simulink model "ImageTest"  (R2015b)
settings: Solver=VariableStepAuto  StartTime=0.0  StopTime=10.0  RelTol=1e-3
undefined symbols (not defined in the file): gray
libraries: visionconversions x1, visionstatistics x1, dspvision x1, visionsinks x1, simulink x1
settings Model: Creator=henry  LastModifiedBy=henry

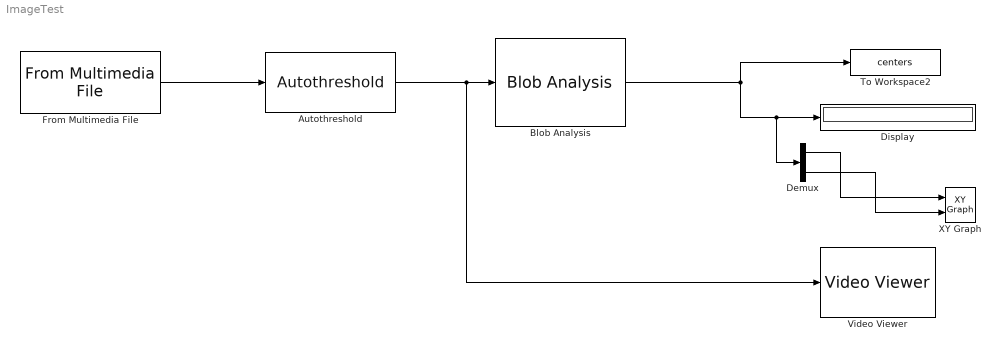
== system ImageTest ==
  Autothreshold : visionconversions/Autothreshold  operator=>  threshOut=off  effMetricOut=off  userDefinedRange=off  umin=0  umax=255  outOfRngOpt=Warn and saturate  scaleThreshold=off  scaleFactor=1  P1Mode=Specify word length  P1WordLength=32  P1FracLength=30  P2Mode=Specify word length  P2WordLength=32  P2FracLength=22  P3Mode=Specify word length  P3WordLength=32  P3FracLength=14  P4Mode=Binary point scaling  P4WordLength=32  P4FracLength=15  Q1Mode=Specify word length  Q1WordLength=32  Q1FracLength=16  EMMode=Specify word length  EMWordLength=16  EMFracLength=14  roundingMode=Floor  overflowMode=off
  Blob Analysis : visionstatistics/Blob Analysis  Tag=vipblks_row_conv  area=off  centroid=on  bBox=off  majorAxis=off  minorAxis=off  angle=off  eccentricity=off  equivDiameterSq=off  extent=off  perimeter=off  maxBlobs=1  warnIfNumBlobsExceeded=off  isCount=off  useMinArea=on  minArea=2000  useMaxArea=on  maxArea=3000  excludeBorderBlob=on  outDT=double  isOutVarDim=off  isFill=off  fillValues=-1  conn=8  isLabel=off  outputMode=Binary point scaling  outputWordLength=32  outputFracLength=16  firstCoeffMode=Binary point scaling  firstCoeffWordLength=16  firstCoeffFracLength=14  secondCoeffMode=Binary point scaling  secondCoeffWordLength=32  secondCoeffFracLength=16  accumMode=Binary point scaling  accumWordLength=32  accumFracLength=0  prodOutputMode=Binary point scaling  prodOutputWordLength=32  prodOutputFracLength=16  roundingMode=Floor  overflowMode=off
  Demux : Demux  Outputs=2
  Display : Display
  From Multimedia File : dspvision/From Multimedia File  inputFilename=/home/henry/MatLab Homework/UH Special Topics/Gitup/MagneticController/Test Videos/output3.ogg  loop=on  numPlays=inf  outputStreams=Video only  videoDataType=single  audioDataType=int16  inheritSampleTime=on  userDefinedSampleTime=1/30  noAudioOutput=off  isIntensityVideo=off  fourcc=Intensity  colorVideoFormat=One multidimensional signal  outputEOF=off  dataOrg=Column-major  audioFrameSize=1024  computeAudioFrameSize=off  outSamplingMode=Sample based
  To Workspace2 : ToWorkspace  VariableName=centers  SampleTime=-1
  Video Viewer : visionsinks/Video Viewer  inputType=Obsolete7b  imagePorts=One multidimensional signal  useColorMap=off  colormapValue=gray(256)  specRange=off  minInputVal=0  maxInputVal=255  FigPos=[181 716 975 554]  AxisZoom=on  trueSizedOnce=off  OpenAtMdlStart=on  DefaultConfigurationName=vipscopes.VideoViewerScopeCfg
  XY Graph : simulink/Sinks/XY Graph  xmin=0  xmax=700  ymin=0  ymax=700  st=-1
  wires:
  Autothreshold/1 -> Video Viewer/1, Blob Analysis/1
  Blob Analysis/1 -> To Workspace2/1, Demux/1, Display/1
  Demux/1 -> XY Graph/1
  Demux/2 -> XY Graph/2
  From Multimedia File/1 -> Autothreshold/1
